simulink model "subtractor"  (R2022b)
settings: Solver=FixedStepAuto  StartTime=0.0  StopTime=inf  RelTol=1e-3
libraries: robotlib x4
settings Model: Creator=sprinkle  LastModifiedBy=sprinkle
settings OptimizationCC: EnhancedBackFolding=on  PassReuseOutputArgsAs=Individual arguments  ZeroExternalMemoryAtStartup=off  ZeroInternalMemoryAtStartup=off  MaxStackSize=64  OptimizeBlockOrder=speed  DifferentSizesBufferReuse=on  OptimizationCustomize=off  EfficientTunableParamExpr=on
settings DebuggingCC: ParameterTunabilityLossMsg=error
settings HardwareCC: ProdBitPerPointer=32  ProdBitPerSizeT=32  ProdBitPerPtrDiffT=32  ProdLargestAtomicFloat=None  ProdIntDivRoundTo=Undefined  ProdEndianess=Unspecified  ProdWordSize=32  ProdHWDeviceType=Generic->Unspecified (assume 32-bit Generic)
settings SFSimCC: MATLABDynamicMemAlloc=off
settings RTWCC: Description=Embedded Coder  SystemTargetFile=ert.tlc  HardwareBoard=Robot Operating System (ROS)  TLCOptions="-aInlineSetEventsForThisBaseRateFcn=TLC_FALSE -aSuppressMultiTaskScheduler=TLC_FALSE  -aRateBasedStepFcn=0"  TemplateMakefile=ert_default_tmf  Toolchain=Catkin  TargetLang=C++
settings CodeAppCC: ForceParamTrailComments=on  IgnoreCustomStorageClasses=off  OperatorAnnotations=on  SimulinkDataObjDesc=on  SFDataObjDesc=on  InsertBlockDesc=on
settings ERTTargetCC: SupportContinuousTime=on

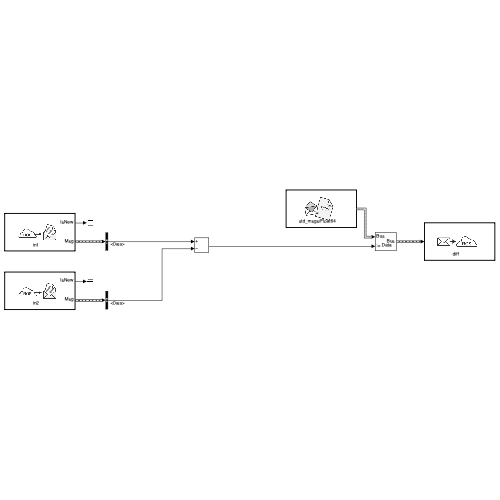
[thumbnail: Simulink's stored preview of the top-level diagram]
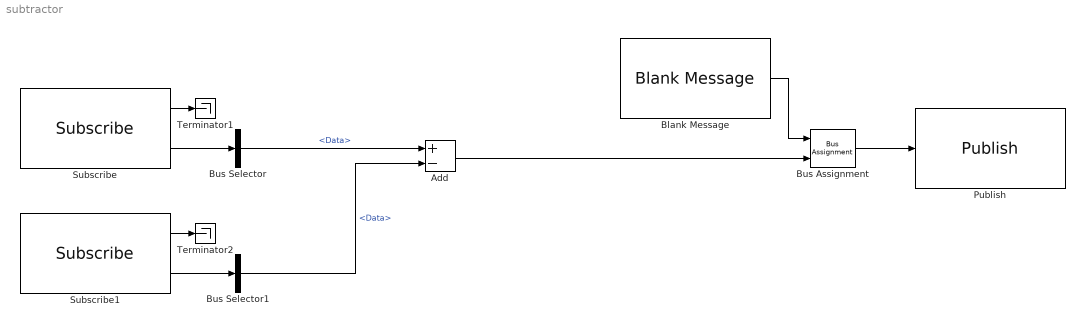
== system subtractor ==
  Add : Sum  Inputs=+-
  Blank Message : robotlib/Blank Message  messageClass=Message  entityType=std_msgs/Float64  messageType=std_msgs/Float64  SampleTime=inf  legacyBusStruct=off
      settings: LibrarySourceBlock=roslib/ROS/Blank Message
  Bus Assignment : BusAssignment  AssignedSignals=Data
  Bus Selector : BusSelector  OutputSignals=Data
  Bus Selector1 : BusSelector  OutputSignals=Data
  Publish : robotlib/Publish  topicSource=Specify your own  topic=diff  messageType=std_msgs/Float64  legacyBusStruct=off  messageQueueLength=1
      settings: LibrarySourceBlock=roslib/ROS/Publish
  Subscribe : robotlib/Subscribe  topicSource=Specify your own  topic=in1  messageType=std_msgs/Float64  SampleTime=-1  legacyBusStruct=off  messageQueueLength=1
      settings: LibrarySourceBlock=roslib/ROS/Subscribe
  Subscribe1 : robotlib/Subscribe  topicSource=Specify your own  topic=in2  messageType=std_msgs/Float64  SampleTime=-1  legacyBusStruct=off  messageQueueLength=1
      settings: LibrarySourceBlock=roslib/ROS/Subscribe
  Terminator1 : Terminator
  Terminator2 : Terminator
  wires:
  Subscribe/2 -> Bus Selector/1
  Bus Selector/1 -> Add/1  "<Data>"
  Blank Message/1 -> Bus Assignment/1
  Bus Assignment/1 -> Publish/1
  Add/1 -> Bus Assignment/2
  Subscribe/1 -> Terminator1/1
  Subscribe1/2 -> Bus Selector1/1
  Bus Selector1/1 -> Add/2  "<Data>"
  Subscribe1/1 -> Terminator2/1
